simulink subsystem "rss_foc_controller_NewPlatform"  (R2023a)
settings: Solver=VariableStepAuto  StartTime=0.0  StopTime=10.0  RelTol=1e-3
undefined symbols (not defined in the file): Cdbl_tiFstTaskSmpTi, Cdbl_tiMedTaskSmpTi, Cdbl_tiSlwTaskSmpTi, ENM_AG_POS_EVAL_MODE, ENM_MOTO_STATUS, ENM_SYS_STATUS
(part 1 of 2)
settings Model: Creator=CAV2OFO  LastModifiedBy=xiaoqiang.yuan
settings SolverCC: AlgebraicLoopSolver=TrustRegion
settings OptimizationCC: ReuseModelBlockBuffer=off
settings DebuggingCC: UnconnectedInputMsg=warning  UnconnectedOutputMsg=warning  UnconnectedLineMsg=warning
settings ModelReferenceCC: EnableRefExpFcnMdlSchedulingChecks=on
settings RTWCC: DLArmComputeVersion=19.05

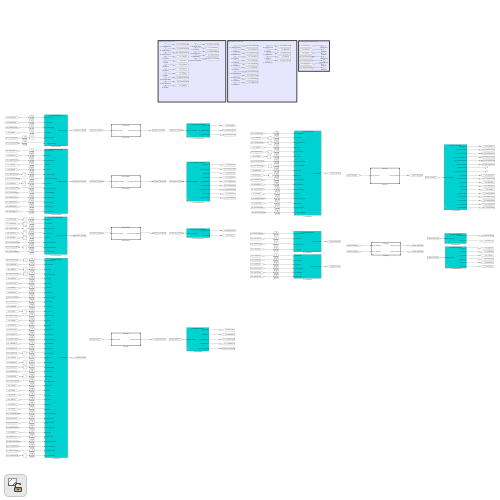
[thumbnail: Simulink's stored preview of the top-level diagram]
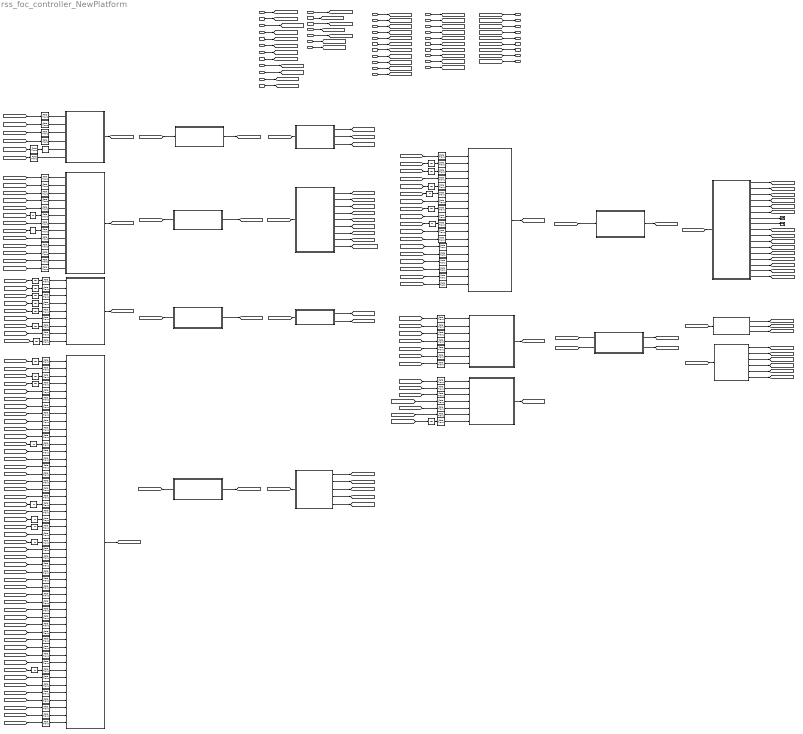
== system rss_foc_controller_NewPlatform ==
  note: Application software signals output
  note: Basic software signals input
  note: Communication signals input
  s16_nComRefMechSpd : Inport  OutDataTypeStr=dt_Standardize_s16p15b0
  u8_modeMCUOpMode : Inport  Port=2  OutDataTypeStr=uint8
  u16_ADSensActMechAg : Inport  Port=3  OutDataTypeStr=uint16
  u16_uADActPhCurr : Inport  Port=4  OutDataTypeStr=uint16
  u16_uADActPhCurrOfs : Inport  Port=5  OutDataTypeStr=uint16
  u8_numSectNum : Inport  Port=6  OutDataTypeStr=uint8
  u16_uADSplyVltg : Inport  Port=7  OutDataTypeStr=uint16
  u16_uADCtlBrdVltg : Inport  Port=8  OutDataTypeStr=uint16
  u16_uADGDVltg : Inport  Port=9  OutDataTypeStr=uint16
  bol_enPosSCDCalibEnFlg : Inport  Port=10  OutDataTypeStr=boolean
  u16_uADPwrTubTemp : Inport  Port=11  OutDataTypeStr=uint16
  u16_uADPCBTemp : Inport  Port=12  OutDataTypeStr=uint16
  u16_uADMotoTemp : Inport  Port=13  OutDataTypeStr=uint16
  u8_ctLossNoData : Inport  Port=14  OutDataTypeStr=uint8
  u8_ctComRolCnt : Inport  Port=15  OutDataTypeStr=uint8
  bol_flgHWOvrCurrFalt : Inport  Port=16  OutDataTypeStr=boolean
  bol_flgChipFalt : Inport  Port=17  OutDataTypeStr=boolean
  bol_flgPhiSensFalt : Inport  Port=18  OutDataTypeStr=boolean
  bol_enFaltInfoClrUDS14 : Inport  Port=19  OutDataTypeStr=boolean
  u16_vVehSpd : Inport  Port=20  OutDataTypeStr=fixdt(0,16,10^-2,0)
  u32_disOde : Inport  Port=21  OutDataTypeStr=fixdt(0,32,10^-1,0)
  u32_tiStamHi : Inport  Port=22  OutDataTypeStr=uint32
  u32_tiStamLo : Inport  Port=23  OutDataTypeStr=uint32
  u8_tOilTemp : Inport  Port=24  OutDataTypeStr=dt_Temp_u8p0bn40
  u8_psiOilFlow : Inport  Port=25  OutDataTypeStr=fixdt(0,8,5^-1,0)
  u8_psiUpLimOilFlow : Inport  Port=26  OutDataTypeStr=fixdt(0,8,5^-1,0)
  bol_flgBusOffFaltRaw : Inport  Port=27  OutDataTypeStr=boolean
  bol_flgFaltEnFlgUDS85 : Inport  Port=28  OutDataTypeStr=boolean
  bol_flgOvrTstCtlUDS2F : Inport  Port=29  OutDataTypeStr=boolean
  bol_flgWBSSt : Inport  Port=30  OutDataTypeStr=boolean
  bol_flgCRCFaltRaw : Inport  Port=31  OutDataTypeStr=boolean
  bol_flgMesgLngthFaltRaw : Inport  Port=32  OutDataTypeStr=boolean
  u8_FrzFrmSaveFlg : Inport  Port=33  OutDataTypeStr=uint8
  bol_flgSlepEn : Inport  Port=34  OutDataTypeStr=boolean
  bol_flgCrashFalt : Inport  Port=35  OutDataTypeStr=boolean
  bol_flgGDVltgHiLvl1 : Inport  Port=36  OutDataTypeStr=boolean
  bol_flgGDVltgLoLvl1 : Inport  Port=37  OutDataTypeStr=boolean
  u8_tMCUTemp : Inport  Port=38  OutDataTypeStr=dt_Temp_u8p0bn40
  u16_phiDvtSensElecAg : Inport  Port=39  OutDataTypeStr=dt_RadAng_u16r15b0
  bol_flgMosOpnCirFalt : Inport  Port=40  OutDataTypeStr=boolean
  ASW_AST : ModelReference  ModelNameDialog=ASW_AST.slx  SimulationMode=Normal  ModelReferenceVersion=6.236
  ASW_DcycGen : ModelReference  ModelNameDialog=ASW_DcycGen.slx  SimulationMode=Normal  ModelReferenceVersion=6.161
  ASW_OBD : ModelReference  ModelNameDialog=ASW_OBD.slx  SimulationMode=Normal  ModelReferenceVersion=6.308
  ASW_PhCurrGen : ModelReference  ModelNameDialog=ASW_PhCurrGen.slx  SimulationMode=Normal  ModelReferenceVersion=6.181
  ASW_PhVltgGen : ModelReference  ModelNameDialog=ASW_PhVltgGen.slx  SimulationMode=Normal  ModelReferenceVersion=6.211
  ASW_SigIn : ModelReference  ModelNameDialog=ASW_SigIn.slx  SimulationMode=Normal  ModelReferenceVersion=6.146
  Delay : Delay  DelayLength=1
  Delay1 : Delay  DelayLength=1
  Rate Transition{1,5..6,8,16,19,22,24..26,29..31,33,36,41,49,109} (18 alike) : RateTransition  Deterministic=off  OutPortSampleTime=round(double(Cdbl_tiMedTaskSmpTi),6)
  Rate Transition{2,9..10,14,48} (5 alike) : RateTransition  Deterministic=off  OutPortSampleTime=round(double(Cdbl_tiFstTaskSmpTi),8)
  Rate Transition100 : RateTransition  Deterministic=off  InitialCondition=ENM_AG_POS_EVAL_MODE.SENSORLESS  OutPortSampleTime=round(double(Cdbl_tiSlwTaskSmpTi),4)
  Rate Transition101 : RateTransition  Deterministic=off  InitialCondition=ENM_AG_POS_EVAL_MODE.SENSOR  OutPortSampleTime=round(double(Cdbl_tiSlwTaskSmpTi),4)
  Rate Transition{3..4,7,15,17..18,20..21,23,27..28,32,34..35,37..40,43..44,46..47,50..99,102..108} (79 alike) : RateTransition  Deterministic=off  OutPortSampleTime=round(double(Cdbl_tiSlwTaskSmpTi),4)
  Rate Transition11 : RateTransition  Deterministic=off  InitialCondition=ENM_MOTO_STATUS.OFF  OutPortSampleTime=round(double(Cdbl_tiFstTaskSmpTi),8)
  Rate Transition12 : RateTransition  Deterministic=off  InitialCondition=ENM_MOTO_STATUS.OFF  OutPortSampleTime=round(double(Cdbl_tiMedTaskSmpTi),6)
  Rate Transition13 : RateTransition  Deterministic=off  InitialCondition=ENM_AG_POS_EVAL_MODE.SENSORLESS  OutPortSampleTime=round(double(Cdbl_tiMedTaskSmpTi),6)
  Rate Transition42 : RateTransition  Deterministic=off  InitialCondition=ENM_MOTO_STATUS.OFF  OutPortSampleTime=round(double(Cdbl_tiSlwTaskSmpTi),4)
  Rate Transition45 : RateTransition  Deterministic=off  InitialCondition=ENM_MOTO_STATUS.OFF  OutPortSampleTime=round(double(Cdbl_tiSlwTaskSmpTi),4)
  Terminator11 : Terminator
  Terminator9 : Terminator
  Unit Delay : UnitDelay  InitialCondition=ENM_AG_POS_EVAL_MODE.SENSOR  SampleTime=-1  HasFrameUpgradeWarning=on
  Unit Delay{1..7,9..18,20..22} (20 alike) : UnitDelay  SampleTime=-1  HasFrameUpgradeWarning=on
  Unit Delay19 : UnitDelay  InitialCondition=ENM_MOTO_STATUS.OFF  SampleTime=-1  HasFrameUpgradeWarning=on
  Unit Delay32 : UnitDelay  InitialCondition=ENM_MOTO_STATUS.OFF  SampleTime=-1  HasFrameUpgradeWarning=on
  Unit Delay8 : UnitDelay  InitialCondition=ENM_SYS_STATUS.SYSINIT  SampleTime=-1  HasFrameUpgradeWarning=on
  sss_SigInSlwTaskIn : Subsystem  VariantControl=cstSenlCtrlLbl
  vrs_ASTSlwTaskIn : Subsystem  Variant=on  VariantControlMode=label  VariantControl=cstSenlCtrlLbl  LabelModeActiveChoice=cstHybrCtrlLbl
  vrs_ASTSlwTaskOut : Subsystem  Variant=on  VariantControlMode=label  VariantControl=Choice  LabelModeActiveChoice=cstHybrCtrlLbl
  vrs_DcycGenFstTaskIn : Subsystem  Variant=on  VariantControlMode=label  VariantControl=Choice  LabelModeActiveChoice=cstSensCtrlLbl
  vrs_DcycGenFstTaskOut : Subsystem  Variant=on  VariantControlMode=label  VariantControl=Choice  LabelModeActiveChoice=cstSensCtrlLbl
  vrs_OBDSlwTaskIn : Subsystem  Variant=on  VariantControlMode=label  VariantControl=cstSenlCtrlLbl  LabelModeActiveChoice=cstHybrCtrlLbl
  vrs_OBDSlwTaskOut : Subsystem  Variant=on  VariantControlMode=label  VariantControl=Choice  LabelModeActiveChoice=cstHybrCtrlLbl
  vrs_PhCurrGenSlwTaskIn : Subsystem  Variant=on  VariantControlMode=label  VariantControl=cstSenlCtrlLbl  LabelModeActiveChoice=cstHybrCtrlLbl
  vrs_PhCurrGenSlwTaskOut : Subsystem  Variant=on  VariantControlMode=label  VariantControl=Choice  LabelModeActiveChoice=cstSenlCtrlLbl
  vrs_PhVltgGenMedTaskIn : Subsystem  Variant=on  VariantControlMode=label  VariantControl=Choice  LabelModeActiveChoice=cstHybrCtrlLbl
  vrs_PhVltgGenMedTaskOut : Subsystem  Variant=on  VariantControlMode=label  VariantControl=Choice  LabelModeActiveChoice=cstHybrCtrlLbl
  vrs_SigInMedTaskIn : Subsystem  Variant=on  VariantControlMode=label  VariantControl=cstSenlCtrlLbl  LabelModeActiveChoice=cstSensCtrlLbl
  vrs_SigInMedTaskOut : Subsystem  Variant=on  VariantControlMode=label  VariantControl=Choice  LabelModeActiveChoice=cstSensCtrlLbl
  vrs_SigInSlwTaskOut : Subsystem  Variant=on  VariantControlMode=label  VariantControl=Choice  LabelModeActiveChoice=cstSenlCtrlLbl
  genXYZDutyCycl : Outport
  enmMotStas : Outport  Port=2
  enmSysStas : Outport  Port=3
  bolCalibSuccFlag : Outport  Port=4
  arSensErrMechAng : Outport  Port=5
  iEstSplyCurr : Outport  Port=6
  iActLineCurr : Outport  Port=7
  u16_phiSensElecAgDvt : Outport  Port=8
  s16_nActElecSpdComFlt : Outport  Port=9
  wires:
  u16_ADSensActMechAg/1 -> [u16_ADSensActMechAg]
  u16_uADActPhCurr/1 -> [u16_uADActPhCurr]
  u16_uADSplyVltg/1 -> [u16_uADSplyVltg]
  [u16_dcycPhDyc] -> genXYZDutyCycl/1
  s16_nComRefMechSpd/1 -> [s16_nComRefMechSpd]
  [s16_iEstSplyCurr] -> iEstSplyCurr/1
  [s16_ampActPhCurrAmp] -> iActLineCurr/1
  [u16_phiModulActElecAg] -> Unit Delay4/1
  [s16_nPredActElecSpd] -> Rate Transition14/1
  [u16_ampDycAmp] -> Rate Transition2/1
  [enm_stMotoSt] -> Rate Transition11/1
  [u16_phiDaxQaxVltgAg] -> Rate Transition10/1
  Rate Transition14/1 -> Delay1/1
  [s16_nActElecSpd] -> Unit Delay5/1
  [s16_nRefElecSpd] -> Unit Delay7/1
  [s16_trqRefTqLim] -> Unit Delay12/1
  [u16_dcycPhDyc] -> Delay/1
  Delay/1 -> Rate Transition31/1
  vrs_PhVltgGenMedTaskIn/1(busPhVltgGen_MedTaskIn) -> [busPhVltgGen_MedTaskIn]
  Rate Transition25/1 -> vrs_PhVltgGenMedTaskIn/1(s16_iRefDaxQaxCurr)
  Rate Transition26/1 -> vrs_PhVltgGenMedTaskIn/2(s16_iActPhCurr)
  Rate Transition1/1 -> vrs_PhVltgGenMedTaskIn/3(u16_phiSensActElecAg)
  Rate Transition6/1 -> vrs_PhVltgGenMedTaskIn/4(u16_uSplyVltg)
  Rate Transition12/1 -> vrs_PhVltgGenMedTaskIn/5(enm_stMotoSt)
  Rate Transition29/1 -> vrs_PhVltgGenMedTaskIn/6(u16_phiModulActElecAg)
  [busPhVltgGen_MedTaskOut] -> vrs_PhVltgGenMedTaskOut/1(busPhVltgGen_MedTaskOut)
  vrs_PhVltgGenMedTaskOut/2(u16_phiDaxQaxVltgAg) -> [u16_phiDaxQaxVltgAg]
  vrs_PhVltgGenMedTaskOut/3(u16_phiActElecAg) -> [u16_phiActElecAg]
  vrs_PhVltgGenMedTaskOut/1(u16_ampDycAmp) -> [u16_ampDycAmp]
  vrs_PhVltgGenMedTaskOut/4(s16_nActElecSpd) -> [s16_nActElecSpd]
  vrs_PhVltgGenMedTaskOut/7(s16_uModulDaxQaxVltg) -> [s16_uModulDaxQaxVltg]
  vrs_PhVltgGenMedTaskOut/5(s16_iActDaxQaxCurr) -> [s16_iActDaxQaxCurr]
  vrs_PhVltgGenMedTaskOut/6(s16_nPredActElecSpd) -> [s16_nPredActElecSpd]
  Rate Transition2/1 -> vrs_DcycGenFstTaskIn/1(u16_ampDycAmp)
  Rate Transition9/1 -> vrs_DcycGenFstTaskIn/2(u16_phiActElecAg)
  Rate Transition10/1 -> vrs_DcycGenFstTaskIn/3(u16_phiDaxQaxVltgAg)
  Rate Transition11/1 -> vrs_DcycGenFstTaskIn/4(enm_stMotoSt)
  Delay1/1 -> vrs_DcycGenFstTaskIn/5(s16_nPredActElecSpd)
  vrs_DcycGenFstTaskIn/1(busDcycGen_FstTaskIn) -> [busDcycGen_FstTaskIn]
  [busDcycGen_FstTaskOut] -> vrs_DcycGenFstTaskOut/1(busDcycGen_FstTaskOut)
  vrs_DcycGenFstTaskOut/1(u16_dcycPhDyc) -> [u16_dcycPhDyc]
  vrs_DcycGenFstTaskOut/2(u16_ampMaxNrmVltgAmp) -> [u16_ampMaxNrmVltgAmp]
  vrs_DcycGenFstTaskOut/3(u16_phiModulActElecAg) -> [u16_phiModulActElecAg]
  vrs_PhCurrGenSlwTaskOut/1(s16_iRefDaxQaxCurr) -> [s16_iRefDaxQaxCurr]
  bol_enPosSCDCalibEnFlg/1 -> [bol_enPosSCDCalibEnFlg]
  Unit Delay4/1 -> Rate Transition29/1
  Unit Delay5/1 -> Rate Transition18/1
  [s16_nRmpRefElecSpd] -> Unit Delay11/1
  [bol_enPosSCDCalibEnFlg] -> Rate Transition39/1
  [bol_flgShOffFlg] -> Unit Delay13/1
  vrs_PhCurrGenSlwTaskOut/2(enm_stMotoSt) -> [enm_stMotoSt]
  vrs_ASTSlwTaskOut/10(s16_nRmpRefElecSpd) -> [s16_nRmpRefElecSpd]
  vrs_ASTSlwTaskOut/3(s16_trqPosSCDCalibRefTq) -> [s16_trqPosSCDCalibRefTq]
  vrs_ASTSlwTaskOut/2(s16_ampActPhCurrAmp) -> [s16_ampActPhCurrAmp]
  vrs_ASTSlwTaskOut/6(u16_ADSensMechAgDvt) -> [u16_ADSensMechAgDvt]
  vrs_ASTSlwTaskOut/8(bol_flgPosSCDCalibPermFail) -> Terminator11/1
  vrs_ASTSlwTaskOut/9(s16_trqRefTqLim) -> [s16_trqRefTqLim]
  vrs_ASTSlwTaskOut/4(u16_phiPosSCDCalibElecAg) -> [u16_phiPosSCDCalibElecAg]
  vrs_ASTSlwTaskOut/5(bol_flgPosSCDCalibSucFlg) -> [bol_flgPosSCDCalibSucFlg]
  vrs_ASTSlwTaskOut/7(enm_stPosSCDCalibSt) -> Terminator9/1
  vrs_ASTSlwTaskOut/1(s16_iEstSplyCurr) -> [s16_iEstSplyCurr]
  [busPhCurrGen_SlwTaskOut] -> vrs_PhCurrGenSlwTaskOut/1(busMotoCtl_SlwTaskOut)
  ASW_AST/1 -> [busAST_SlwTaskOut]
  [busAST_SlwTaskIn] -> ASW_AST/1
  [busAST_SlwTaskOut] -> vrs_ASTSlwTaskOut/1(busAST_SlwTaskOut)
  [s16_iActDaxQaxCurr] -> Unit Delay9/1
  [s16_uModulDaxQaxVltg] -> Unit Delay10/1
  [s16_nComRefMechSpd] -> Rate Transition4/1
  [s16_nActElecSpd] -> Unit Delay6/1
  Unit Delay6/1 -> Rate Transition15/1
  Unit Delay9/1 -> Rate Transition40/1
  Unit Delay10/1 -> Rate Transition23/1
  Unit Delay11/1 -> Rate Transition20/1
  Unit Delay12/1 -> Rate Transition21/1
  [s16_nRmpRefElecSpd] -> Unit Delay3/1
  [busOBD_SlwTaskIn] -> ASW_OBD/1
  [enm_stMotoSt] -> Unit Delay19/1
  [s16_nActElecSpd] -> Rate Transition44/1
  [busOBD_SlwTaskOut] -> vrs_OBDSlwTaskOut/1(busOBD_SlwTaskOut)
  ASW_OBD/1 -> [busOBD_SlwTaskOut]
  vrs_SigInMedTaskOut/1(u16_phiSensActElecAg) -> [u16_phiSensActElecAg]
  ASW_SigIn/1 -> [busSigIn_MedTaskOut]
  [busSigIn_MedTaskOut] -> vrs_SigInMedTaskOut/1(busSigIn_MedTaskOut)
  [busSigIn_MedTaskIn] -> ASW_SigIn/1
  [u16_ADSensActMechAg] -> Rate Transition49/1
  vrs_ASTSlwTaskOut/11(bol_flgShOffFlg) -> [bol_flgShOffFlg]
  Unit Delay13/1 -> Rate Transition38/1
  [bol_enPosSCDCalibEnFlg] -> Rate Transition48/1
  [u16_phiSensActElecAg] -> Unit Delay15/1
  Unit Delay15/1 -> Rate Transition51/1
  Rate Transition36/1 -> vrs_PhVltgGenMedTaskIn/7(u16_phiPosSCDCalibElecAg)
  Rate Transition31/1 -> vrs_PhVltgGenMedTaskIn/8(u16_dcycPhDyc)
  Rate Transition41/1 -> vrs_PhVltgGenMedTaskIn/9(bol_enPosSCDCalibEnFlg)
  Rate Transition13/1 -> vrs_PhVltgGenMedTaskIn/10(enm_modeAgEvalMode)
  Rate Transition33/1 -> vrs_PhVltgGenMedTaskIn/11(s16_nRmpRefElecSpd)
  [s16_trqPosSCDCalibRefTq] -> Unit Delay16/1
  Unit Delay16/1 -> Rate Transition53/1
  vrs_ASTSlwTaskOut/12(s16_nRefElecSpd) -> [s16_nRefElecSpd]
  [enm_stMotoSt] -> Unit Delay32/1
  Unit Delay7/1 -> Rate Transition17/1
  u16_uADPwrTubTemp/1 -> [u16_uADPwrTubTemp]
  u16_uADPCBTemp/1 -> [u16_uADPCBTemp]
  u16_uADMotoTemp/1 -> [u16_uADMotoTemp]
  u8_ctLossNoData/1 -> [u8_ctLossNoData]
  u8_ctComRolCnt/1 -> [u8_ctComRolCnt]
  u8_modeMCUOpMode/1 -> [u8_modeMCUOpMode]
  [u16_uADActPhCurr] -> Rate Transition22/1
  [u16_uADPwrTubTemp] -> Rate Transition61/1
  [u16_uADPCBTemp] -> Rate Transition62/1
  [u16_uADMotoTemp] -> Rate Transition63/1
  Rate Transition61/1 -> sss_SigInSlwTaskIn/3(u16_uADPwrTubTemp)
  Rate Transition62/1 -> sss_SigInSlwTaskIn/4(u16_uADPCBTemp)
  Rate Transition63/1 -> sss_SigInSlwTaskIn/5(u16_uADMotoTemp)
  sss_SigInSlwTaskIn/1(busSigIn_SlowTaskInp) -> [busSigIn_SlwTaskIn]
  [busSigIn_SlwTaskIn] -> ASW_SigIn/2
  ASW_SigIn/2 -> [busSigIn_SlwTaskOut]
  vrs_SigInMedTaskOut/2(s16_iActPhCurr) -> [s16_iActPhCurr]
  [busSigIn_SlwTaskOut] -> vrs_SigInSlwTaskOut/1(busSigIn_SlwTaskOut)
  vrs_SigInSlwTaskOut/4(u8_tPCBTemp) -> [u8_tPCBTemp]
  vrs_SigInSlwTaskOut/5(u8_tMotoTemp) -> [u8_tMotoTemp]
  vrs_OBDSlwTaskOut/1(busOBD_FaltSt) -> [busOBD_FaltSt]
  vrs_OBDSlwTaskOut/2(u8_stMaxFaltLvl) -> [u8_stMaxFaltLvl]
  vrs_OBDSlwTaskOut/3(s16_nFaltRefMechSpd) -> [s16_nFaltRefMechSpd]
  vrs_OBDSlwTaskOut/4(s16_trqFaltRefTqLim) -> [s16_trqFaltRefTqLim]
  [s16_ampActPhCurrAmp] -> Unit Delay17/1
  [u16_uSplyVltg] -> Rate Transition65/1
  [u8_tPwrTubTemp] -> Rate Transition66/1
  [u8_tPCBTemp] -> Rate Transition67/1
  [u8_tMotoTemp] -> Rate Transition68/1
  [u8_ctLossNoData] -> Rate Transition69/1
  [u8_ctComRolCnt] -> Rate Transition70/1
  vrs_ASTSlwTaskOut/13(enm_stSysSt) -> [enm_stSysSt]
  [busOBD_FaltSt] -> Unit Delay1/1
  Unit Delay1/1 -> Rate Transition73/1
  Unit Delay3/1 -> Rate Transition43/1
  Unit Delay17/1 -> Rate Transition64/1
  [enm_stMotoSt] -> enmMotStas/1
  [enm_stSysSt] -> enmSysStas/1
  [bol_flgPosSCDCalibSucFlg] -> bolCalibSuccFlag/1
  [u16_ADSensMechAgDvt] -> arSensErrMechAng/1
  [s16_nRmpRefElecSpd] -> Rate Transition33/1
  Rate Transition19/1 -> vrs_PhVltgGenMedTaskIn/13(u16_ampMaxNrmVltgAmp)
  [u16_uADActPhCurrOfs] -> Rate Transition24/1
  [u8_numSectNum] -> Rate Transition30/1
  u16_uADActPhCurrOfs/1 -> [u16_uADActPhCurrOfs]
  u8_numSectNum/1 -> [u8_numSectNum]
  vrs_SigInSlwTaskOut/3(u8_tPwrTubTemp) -> [u8_tPwrTubTemp]
  [u16_phiActElecAg] -> Rate Transition9/1
  [u16_uCtlBrdVltg] -> Rate Transition27/1
  vrs_SigInSlwTaskOut/1(u16_uCtlBrdVltg) -> [u16_uCtlBrdVltg]
  Rate Transition28/1 -> sss_SigInSlwTaskIn/1(u16_uADCtlBrdVltg)
  [u16_uADCtlBrdVltg] -> Rate Transition28/1
  u16_uADCtlBrdVltg/1 -> [u16_uADCtlBrdVltg]
  [busDcycGen_FstTaskIn] -> ASW_DcycGen/1
  [busPhVltgGen_MedTaskIn] -> ASW_PhVltgGen/1
  [busPhCurrGen_SlwTaskIn] -> ASW_PhCurrGen/1
  ASW_DcycGen/1 -> [busDcycGen_FstTaskOut]
  ASW_PhVltgGen/1 -> [busPhVltgGen_MedTaskOut]
  ASW_PhCurrGen/1 -> [busPhCurrGen_SlwTaskOut]
  u16_uADGDVltg/1 -> [u16_uADGDVltg]
  Rate Transition32/1 -> sss_SigInSlwTaskIn/2(u16_uADGDVltg)
  [u16_uADGDVltg] -> Rate Transition32/1
  vrs_SigInSlwTaskOut/2(u16_uGDVltg) -> [u16_uGDVltg]
  [enm_stSysSt] -> Unit Delay8/1
  [bol_flgHWOvrCurrFalt] -> Rate Transition46/1
  [bol_flgChipFalt] -> Rate Transition52/1
  [bol_flgPhiSensFalt] -> Rate Transition54/1
  [u16_uADActPhCurr] -> Rate Transition55/1
  [u16_uADPwrTubTemp] -> Rate Transition56/1
  [u16_uADPCBTemp] -> Rate Transition57/1
  [u16_uADMotoTemp] -> Rate Transition58/1
  [s16_pwrSplyElecPwr] -> Unit Delay2/1
  bol_flgHWOvrCurrFalt/1 -> [bol_flgHWOvrCurrFalt]
  bol_flgChipFalt/1 -> [bol_flgChipFalt]
  bol_flgPhiSensFalt/1 -> [bol_flgPhiSensFalt]
  vrs_ASTSlwTaskOut/14(s16_pwrSplyElecPwr) -> [s16_pwrSplyElecPwr]
  Unit Delay2/1 -> Rate Transition59/1
  Unit Delay8/1 -> Rate Transition34/1
  [s16_iActPhCurr] -> Rate Transition60/1
  [s16_iEstSplyCurr] -> Unit Delay14/1
  [s16_iRefDaxQaxCurr] -> Unit Delay20/1
  [s16_iActDaxQaxCurr] -> Rate Transition81/1
  [bol_flgShOffFlg] -> Unit Delay18/1
  Unit Delay14/1 -> Rate Transition71/1
  Unit Delay18/1 -> Rate Transition82/1
  [bol_enFaltInfoClrUDS14] -> Rate Transition83/1
  [u16_vVehSpd] -> Rate Transition84/1
  [u32_disOde] -> Rate Transition85/1
  [u32_tiStamHi] -> Rate Transition86/1
  [u32_tiStamLo] -> Rate Transition87/1
  [u8_psiOilFlow] -> Rate Transition88/1
  [u8_tOilTemp] -> Rate Transition89/1
  [bol_enPosSCDCalibEnFlg] -> Rate Transition90/1
  [u8_psiUpLimOilFlow] -> Rate Transition91/1
  bol_enFaltInfoClrUDS14/1 -> [bol_enFaltInfoClrUDS14]
  u16_vVehSpd/1 -> [u16_vVehSpd]
  u32_disOde/1 -> [u32_disOde]
  u32_tiStamHi/1 -> [u32_tiStamHi]
  u32_tiStamLo/1 -> [u32_tiStamLo]
  u8_tOilTemp/1 -> [u8_tOilTemp]
  u8_psiOilFlow/1 -> [u8_psiOilFlow]
  u8_psiUpLimOilFlow/1 -> [u8_psiUpLimOilFlow]
  bol_flgBusOffFaltRaw/1 -> [bol_flgBusOffFaltRaw]
  bol_flgFaltEnFlgUDS85/1 -> [bol_flgFaltEnFlgUDS85]
  bol_flgOvrTstCtlUDS2F/1 -> [bol_flgOvrTstCtlUDS2F]
  bol_flgWBSSt/1 -> [bol_flgWBSSt]
  [bol_flgBusOffFaltRaw] -> Rate Transition93/1
  [bol_flgFaltEnFlgUDS85] -> Rate Transition94/1
  [bol_flgWBSSt] -> Rate Transition95/1
  bol_flgCRCFaltRaw/1 -> [bol_flgCRCFaltRaw]
  bol_flgMesgLngthFaltRaw/1 -> [bol_flgMesgLngthFaltRaw]
  [bol_flgCRCFaltRaw] -> Rate Transition96/1
  [bol_flgMesgLngthFaltRaw] -> Rate Transition97/1
  [s16_nComRefMechSpd] -> Rate Transition98/1
  vrs_PhVltgGenMedTaskOut/8(u16_psiEstPermMagFlx) -> [u16_psiEstPermMagFlx]
  [u16_psiEstPermMagFlx] -> Rate Transition99/1
  Rate Transition43/1 -> vrs_OBDSlwTaskIn/1(s16_nRmpRefElecSpd)
  Rate Transition44/1 -> vrs_OBDSlwTaskIn/2(s16_nActElecSpd)
  Rate Transition45/1 -> vrs_OBDSlwTaskIn/3(enm_stMotoSt)
  Rate Transition64/1 -> vrs_OBDSlwTaskIn/4(s16_ampActPhCurrAmp)
  Rate Transition65/1 -> vrs_OBDSlwTaskIn/5(u16_uSplyVltg)
  Rate Transition66/1 -> vrs_OBDSlwTaskIn/6(u8_tPwrTubTemp)
  Rate Transition67/1 -> vrs_OBDSlwTaskIn/7(u8_tPCBTemp)
  Rate Transition68/1 -> vrs_OBDSlwTaskIn/8(u8_tMotoTemp)
  Rate Transition69/1 -> vrs_OBDSlwTaskIn/9(u8_ctLossNoData)
  Rate Transition70/1 -> vrs_OBDSlwTaskIn/10(u8_ctComRolCnt)
  Rate Transition27/1 -> vrs_OBDSlwTaskIn/11(u16_uCtlBrdVltg)
  Rate Transition34/1 -> vrs_OBDSlwTaskIn/12(enm_stSysSt)
  Rate Transition46/1 -> vrs_OBDSlwTaskIn/13(bol_flgHWOvrCurrFalt)
  Rate Transition52/1 -> vrs_OBDSlwTaskIn/14(bol_flgChipFalt)
  Rate Transition54/1 -> vrs_OBDSlwTaskIn/15(bol_flgPhiSensFalt)
  Rate Transition55/1 -> vrs_OBDSlwTaskIn/16(u16_uADActPhCurr)
  Rate Transition56/1 -> vrs_OBDSlwTaskIn/17(u16_uADPwrTubTemp)
  Rate Transition57/1 -> vrs_OBDSlwTaskIn/18(u16_uADPCBTemp)
  Rate Transition58/1 -> vrs_OBDSlwTaskIn/19(u16_uADMotoTemp)
  Rate Transition59/1 -> vrs_OBDSlwTaskIn/20(s16_pwrSplyElecPwr)
  Rate Transition60/1 -> vrs_OBDSlwTaskIn/21(s16_iActPhCurr)
  Rate Transition71/1 -> vrs_OBDSlwTaskIn/22(s16_iEstSplyCurr)
  Rate Transition80/1 -> vrs_OBDSlwTaskIn/23(s16_iRefDaxQaxCurr)
  Rate Transition81/1 -> vrs_OBDSlwTaskIn/24(s16_iActDaxQaxCurr)
  Rate Transition82/1 -> vrs_OBDSlwTaskIn/25(bol_flgShOffFlg)
  Rate Transition83/1 -> vrs_OBDSlwTaskIn/26(bol_enFaltInfoClrUDS14)
  Rate Transition84/1 -> vrs_OBDSlwTaskIn/27(u16_vVehSpd)
  Rate Transition85/1 -> vrs_OBDSlwTaskIn/28(u32_disOde)
  Rate Transition86/1 -> vrs_OBDSlwTaskIn/29(u32_tiStamHi)
  Rate Transition87/1 -> vrs_OBDSlwTaskIn/30(u32_tiStamLo)
  Rate Transition88/1 -> vrs_OBDSlwTaskIn/31(u8_psiOilFlow)
  Rate Transition89/1 -> vrs_OBDSlwTaskIn/32(u8_tOilTemp)
  Rate Transition90/1 -> vrs_OBDSlwTaskIn/33(bol_enPosSCDCalibEnFlg)
  Rate Transition91/1 -> vrs_OBDSlwTaskIn/34(u8_psiUpLimOilFlow)
  Rate Transition93/1 -> vrs_OBDSlwTaskIn/35(bol_flgBusOffFaltRaw)
  Rate Transition94/1 -> vrs_OBDSlwTaskIn/36(bol_flgFaltEnFlgUDS85)
  Rate Transition95/1 -> vrs_OBDSlwTaskIn/37(bol_flgWBSSt)
  Rate Transition96/1 -> vrs_OBDSlwTaskIn/38(bol_flgCRCFaltRaw)
  Rate Transition97/1 -> vrs_OBDSlwTaskIn/39(bol_flgMesgLngthFaltRaw)
  Rate Transition98/1 -> vrs_OBDSlwTaskIn/40(s16_nComRefMechSpd)
  Rate Transition99/1 -> vrs_OBDSlwTaskIn/41(u16_psiEstPermMagFlx)
  vrs_OBDSlwTaskIn/1(busSlowTaskInp) -> [busOBD_SlwTaskIn]
  Rate Transition49/1 -> vrs_SigInMedTaskIn/1(u16_ADSensActMechAg)
  Rate Transition22/1 -> vrs_SigInMedTaskIn/2(u16_uADActPhCurr)
  Rate Transition24/1 -> vrs_SigInMedTaskIn/3(u16_uADActPhCurrOfs)
  Rate Transition30/1 -> vrs_SigInMedTaskIn/4(u8_numSectNum)
  vrs_SigInMedTaskIn/1(busSigIn_MedTaskIn) -> [busSigIn_MedTaskIn]
  vrs_ASTSlwTaskOut/15(enm_modeAgEvalMode) -> [enm_modeAgEvalMode]
  Rate Transition17/1 -> vrs_PhCurrGenSlwTaskIn/1(s16_nRefElecSpd)
  Rate Transition18/1 -> vrs_PhCurrGenSlwTaskIn/2(s16_nActElecSpd)
  Rate Transition20/1 -> vrs_PhCurrGenSlwTaskIn/3(s16_nRmpRefElecSpd)
  Rate Transition21/1 -> vrs_PhCurrGenSlwTaskIn/4(s16_trqRefTqLim)
  Rate Transition38/1 -> vrs_PhCurrGenSlwTaskIn/5(bol_flgShOffFlg)
  Rate Transition39/1 -> vrs_PhCurrGenSlwTaskIn/6(bol_enPosSCDCalibEnFlg)
  Rate Transition53/1 -> vrs_PhCurrGenSlwTaskIn/7(s16_trqPosSCDCalibRefTq)
  vrs_PhCurrGenSlwTaskIn/1(busPhCurrGen_SlwTaskIn) -> [busPhCurrGen_SlwTaskIn]
  Rate Transition4/1 -> vrs_ASTSlwTaskIn/1(s16_nComRefMechSpd)
  Rate Transition15/1 -> vrs_ASTSlwTaskIn/2(s16_nActElecSpd)
  Rate Transition23/1 -> vrs_ASTSlwTaskIn/3(s16_uModulDaxQaxVltg)
  Rate Transition37/1 -> vrs_ASTSlwTaskIn/4(u16_uSplyVltg)
  Rate Transition40/1 -> vrs_ASTSlwTaskIn/5(s16_iActDaxQaxCurr)
  Rate Transition42/1 -> vrs_ASTSlwTaskIn/6(enm_stMotoSt)
  Rate Transition47/1 -> vrs_ASTSlwTaskIn/7(bol_enPosSCDCalibEnFlg)
  Rate Transition51/1 -> vrs_ASTSlwTaskIn/8(u16_phiSensActElecAg)
  Rate Transition72/1 -> vrs_ASTSlwTaskIn/9(u8_stMaxFaltLvl)
  Rate Transition73/1 -> vrs_ASTSlwTaskIn/10(busOBD_FaltSt)
  Rate Transition74/1 -> vrs_ASTSlwTaskIn/11(s16_nFaltRefMechSpd)
  Rate Transition75/1 -> vrs_ASTSlwTaskIn/12(s16_trqFaltRefTqLim)
  Rate Transition79/1 -> vrs_ASTSlwTaskIn/13(u8_modeMCUOpMode)
  Rate Transition3/1 -> vrs_ASTSlwTaskIn/14(u8_tPCBTempSubs)
  Rate Transition92/1 -> vrs_ASTSlwTaskIn/15(bol_flgOvrTstCtlUDS2F)
  vrs_ASTSlwTaskIn/1(busAST_SlwTaskIn) -> [busAST_SlwTaskIn]
  Rate Transition100/1 -> vrs_PhCurrGenSlwTaskIn/8(enm_modeAgEvalMode)
  [enm_modeAgEvalMode] -> Rate Transition100/1
  Rate Transition101/1 -> vrs_OBDSlwTaskIn/42(enm_modeAgEvalMode)
  [enm_modeAgEvalMode] -> Unit Delay/1
  vrs_OBDSlwTaskOut/5(bol_flgPhiSensFaltRawFlg) -> [bol_flgPhiSensFaltRawFlg]
  Rate Transition102/1 -> vrs_ASTSlwTaskIn/16(bol_flgPhiSensFaltRawFlg)
  Unit Delay/1 -> Rate Transition101/1
  Rate Transition48/1 -> vrs_DcycGenFstTaskIn/6(bol_enPosSCDCalibEnFlg)
  [bol_enPosSCDCalibEnFlg] -> Rate Transition41/1
  [u16_phiPosSCDCalibElecAg] -> Rate Transition36/1
  [enm_stMotoSt] -> Rate Transition12/1
  [u16_uSplyVltg] -> Rate Transition6/1
  [u16_phiSensActElecAg] -> Rate Transition1/1
  [s16_iActPhCurr] -> Rate Transition26/1
  [s16_iRefDaxQaxCurr] -> Rate Transition25/1
  [enm_modeAgEvalMode] -> Rate Transition13/1
  [u16_uSplyVltg] -> Rate Transition37/1
  Unit Delay32/1 -> Rate Transition42/1
  [bol_enPosSCDCalibEnFlg] -> Rate Transition47/1
  [u8_stMaxFaltLvl] -> Rate Transition72/1
  [s16_nFaltRefMechSpd] -> Rate Transition74/1
  [s16_trqFaltRefTqLim] -> Rate Transition75/1
  [u8_modeMCUOpMode] -> Rate Transition79/1
  [u8_tPCBTempSubs] -> Rate Transition3/1
  [bol_flgOvrTstCtlUDS2F] -> Rate Transition92/1
  [bol_flgPhiSensFaltRawFlg] -> Rate Transition102/1
  Unit Delay19/1 -> Rate Transition45/1
  Unit Delay20/1 -> Rate Transition80/1
  [u8_FrzFrmSaveFlg] -> Rate Transition76/1
  Rate Transition76/1 -> vrs_ASTSlwTaskIn/17(u8_FrzFrmSaveFlg)
  u8_FrzFrmSaveFlg/1 -> [u8_FrzFrmSaveFlg]
  [bol_flgSlepEn] -> Rate Transition77/1
  Rate Transition77/1 -> vrs_ASTSlwTaskIn/18(bol_flgSlepEn)
  bol_flgSlepEn/1 -> [bol_flgSlepEn]
  [bol_flgCrashFalt] -> Rate Transition78/1
  Rate Transition78/1 -> vrs_OBDSlwTaskIn/43(bol_flgCrashFalt)
  [bol_flgGDVltgHiLvl1] -> Rate Transition103/1
  Rate Transition103/1 -> vrs_OBDSlwTaskIn/44(bol_flgGDVltgHiLvl1)
  Rate Transition104/1 -> vrs_OBDSlwTaskIn/45(bol_flgGDVltgLoLvl1)
  [bol_flgGDVltgLoLvl1] -> Rate Transition104/1
  bol_flgCrashFalt/1 -> [bol_flgCrashFalt]
  bol_flgGDVltgHiLvl1/1 -> [bol_flgGDVltgHiLvl1]
  bol_flgGDVltgLoLvl1/1 -> [bol_flgGDVltgLoLvl1]
  [u8_tMCUTemp] -> Rate Transition50/1
  Rate Transition50/1 -> vrs_OBDSlwTaskIn/46(u8_tMCUTemp)
  u8_tMCUTemp/1 -> [u8_tMCUTemp]
  [u8_tMCUTemp] -> Rate Transition105/1
  Unit Delay21/1 -> Rate Transition106/1
  [busOBD_FaltSt] -> Unit Delay21/1
  Rate Transition105/1 -> sss_SigInSlwTaskIn/6(u8_tMCUTemp)
  Rate Transition106/1 -> sss_SigInSlwTaskIn/7(busOBD_FaltSt)
  vrs_SigInSlwTaskOut/6(u8_tPCBTempSubs) -> [u8_tPCBTempSubs]
  [u8_tPCBTempSubs] -> Rate Transition107/1
  Rate Transition107/1 -> vrs_OBDSlwTaskIn/47(u8_tPCBTempSubs)
  [u16_uGDVltg] -> Rate Transition108/1
  Rate Transition108/1 -> vrs_OBDSlwTaskIn/48(u16_uGDVltg)
  [u8_tPCBTempSubs] -> Rate Transition109/1
  Rate Transition109/1 -> vrs_PhVltgGenMedTaskIn/12(u8_tPCBTempSubs)
  [u16_ampMaxNrmVltgAmp] -> Rate Transition19/1
  vrs_SigInMedTaskOut/3(u16_uSplyVltg) -> [u16_uSplyVltg]
  Rate Transition5/1 -> vrs_SigInMedTaskIn/5(u16_uADSplyVltg)
  [u16_uADSplyVltg] -> Rate Transition5/1
  vrs_PhVltgGenMedTaskOut/9(s16_phiOpnLpAgClsLpAgDvt) -> [s16_phiOpnLpAgClsLpAgDvt]
  Rate Transition7/1 -> vrs_PhCurrGenSlwTaskIn/9(s16_phiOpnLpAgClsLpAgDvt)
  [s16_phiOpnLpAgClsLpAgDvt] -> Unit Delay22/1
  Unit Delay22/1 -> Rate Transition7/1
  vrs_ASTSlwTaskOut/16(u16_phiSensElecAgDvt) -> [u16_phiSensElecAgDvt]
  [u16_phiSensElecAgDvt] -> u16_phiSensElecAgDvt/1
  vrs_ASTSlwTaskOut/17(s16_nActElecSpdComFlt) -> [s16_nActElecSpdComFlt]
  [s16_nActElecSpdComFlt] -> s16_nActElecSpdComFlt/1
  Rate Transition8/1 -> vrs_SigInMedTaskIn/6(u16_phiDvtSensElecAg)
  [u16_phiDvtSensElecAg] -> Rate Transition8/1
  Rate Transition16/1 -> vrs_SigInMedTaskIn/7(bol_enPosSCDCalibEnFlg)
  [bol_enPosSCDCalibEnFlg] -> Rate Transition16/1
  u16_phiDvtSensElecAg/1 -> [u16_phiDvtSensElecAg]
  [bol_flgMosOpnCirFalt] -> Rate Transition35/1
  Rate Transition35/1 -> vrs_OBDSlwTaskIn/49(bol_flgMosOpnCirFalt)
  bol_flgMosOpnCirFalt/1 -> [bol_flgMosOpnCirFalt]

== system rss_foc_controller_NewPlatform/sss_SigInSlwTaskIn ==
  u16_uADCtlBrdVltg : Inport
  u16_uADGDVltg : Inport  Port=2
  u16_uADPwrTubTemp : Inport  Port=3
  u16_uADPCBTemp : Inport  Port=4
  u16_uADMotoTemp : Inport  Port=5
  u8_tMCUTemp : Inport  Port=6
  busOBD_FaltSt : Inport  Port=7
  Bus Creator : BusCreator  Inputs=7  OutDataTypeStr=Bus: BUS_SIGIN_SLW_TASK_IN
      settings: InheritFromInputs=off
  busSigIn_SlowTaskInp : Outport  OutDataTypeStr=Bus: BUS_SIGIN_SLW_TASK_IN
  wires:
  busOBD_FaltSt/1 -> Bus Creator/7
  u8_tMCUTemp/1 -> Bus Creator/6
  u16_uADMotoTemp/1 -> Bus Creator/5
  u16_uADPCBTemp/1 -> Bus Creator/4
  u16_uADPwrTubTemp/1 -> Bus Creator/3
  u16_uADGDVltg/1 -> Bus Creator/2
  u16_uADCtlBrdVltg/1 -> Bus Creator/1
  Bus Creator/1 -> busSigIn_SlowTaskInp/1

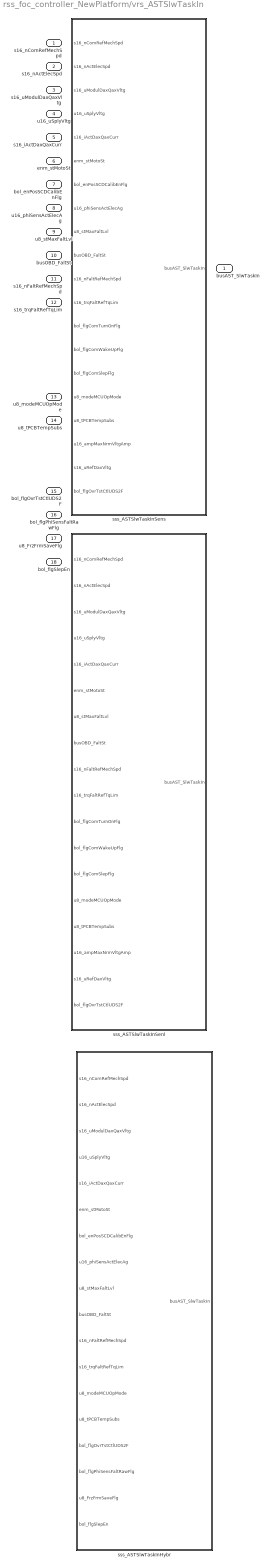
== system rss_foc_controller_NewPlatform/vrs_ASTSlwTaskIn ==
  s16_nComRefMechSpd : Inport
  s16_nActElecSpd : Inport  Port=2
  s16_uModulDaxQaxVltg : Inport  Port=3
  u16_uSplyVltg : Inport  Port=4
  s16_iActDaxQaxCurr : Inport  Port=5
  enm_stMotoSt : Inport  Port=6
  bol_enPosSCDCalibEnFlg : Inport  Port=7
  u16_phiSensActElecAg : Inport  Port=8
  u8_stMaxFaltLvl : Inport  Port=9
  busOBD_FaltSt : Inport  Port=10
  s16_nFaltRefMechSpd : Inport  Port=11
  s16_trqFaltRefTqLim : Inport  Port=12
  u8_modeMCUOpMode : Inport  Port=13
  u8_tPCBTempSubs : Inport  Port=14
  bol_flgOvrTstCtlUDS2F : Inport  Port=15
  bol_flgPhiSensFaltRawFlg : Inport  Port=16
  u8_FrzFrmSaveFlg : Inport  Port=17
  bol_flgSlepEn : Inport  Port=18
  sss_ASTSlwTaskInHybr : Subsystem  VariantControl=cstHybrCtrlLbl
  sss_ASTSlwTaskInSenl : Subsystem  VariantControl=cstSenlCtrlLbl
  sss_ASTSlwTaskInSens : Subsystem  VariantControl=cstSensCtrlLbl
  busAST_SlwTaskIn : Outport

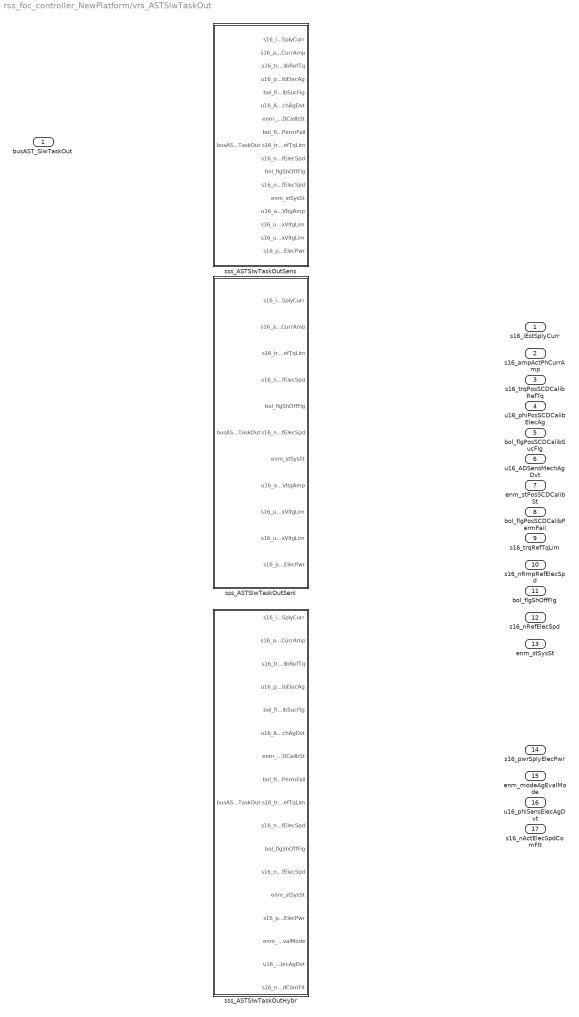
== system rss_foc_controller_NewPlatform/vrs_ASTSlwTaskOut ==
  busAST_SlwTaskOut : Inport
  sss_ASTSlwTaskOutHybr : Subsystem  VariantControl=cstHybrCtrlLbl
  sss_ASTSlwTaskOutSenl : Subsystem  VariantControl=cstSenlCtrlLbl
  sss_ASTSlwTaskOutSens : Subsystem  VariantControl=cstSensCtrlLbl
  s16_iEstSplyCurr : Outport
  s16_ampActPhCurrAmp : Outport  Port=2
  s16_trqPosSCDCalibRefTq : Outport  Port=3
  u16_phiPosSCDCalibElecAg : Outport  Port=4
  bol_flgPosSCDCalibSucFlg : Outport  Port=5
  u16_ADSensMechAgDvt : Outport  Port=6
  enm_stPosSCDCalibSt : Outport  Port=7
  bol_flgPosSCDCalibPermFail : Outport  Port=8
  s16_trqRefTqLim : Outport  Port=9
  s16_nRmpRefElecSpd : Outport  Port=10
  bol_flgShOffFlg : Outport  Port=11
  s16_nRefElecSpd : Outport  Port=12
  enm_stSysSt : Outport  Port=13
  s16_pwrSplyElecPwr : Outport  Port=14
  enm_modeAgEvalMode : Outport  Port=15
  u16_phiSensElecAgDvt : Outport  Port=16
  s16_nActElecSpdComFlt : Outport  Port=17

== system rss_foc_controller_NewPlatform/vrs_DcycGenFstTaskIn ==
  u16_ampDycAmp : Inport
  u16_phiActElecAg : Inport  Port=2
  u16_phiDaxQaxVltgAg : Inport  Port=3
  enm_stMotoSt : Inport  Port=4
  s16_nPredActElecSpd : Inport  Port=5
  bol_enPosSCDCalibEnFlg : Inport  Port=6
  sss_DcycGenFstTaskInSenl : Subsystem  VariantControl=cstSenlCtrlLbl
  sss_DcycGenFstTaskInSens : Subsystem  VariantControl=cstSensCtrlLbl
  busDcycGen_FstTaskIn : Outport  OutDataTypeStr=Bus: BUS_DCYCGEN_FST_TASK_IN

== system rss_foc_controller_NewPlatform/vrs_DcycGenFstTaskOut ==
  busDcycGen_FstTaskOut : Inport
  sss_DcycGenFstTaskOutSenl : Subsystem  VariantControl=cstSenlCtrlLbl
  sss_DcycGenFstTaskOutSens : Subsystem  VariantControl=cstSensCtrlLbl
  u16_dcycPhDyc : Outport  OutDataTypeStr=dt_DutyCycl_u16p15b0
  u16_ampMaxNrmVltgAmp : Outport  Port=2  OutDataTypeStr=dt_DutyCycl_u16p15b0
  u16_phiModulActElecAg : Outport  Port=3  OutDataTypeStr=dt_RadAng_u16r15b0

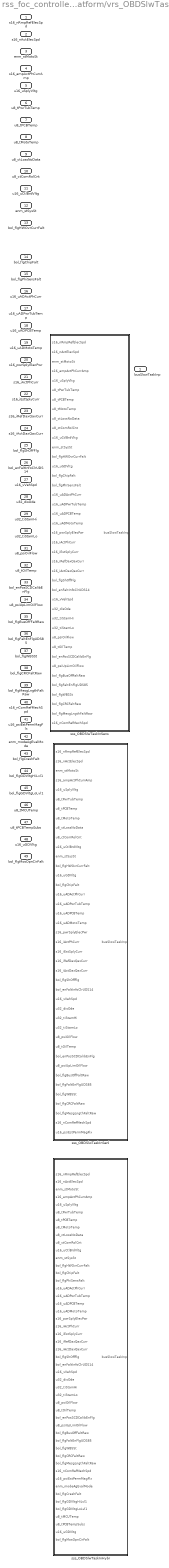
== system rss_foc_controller_NewPlatform/vrs_OBDSlwTaskIn ==
  s16_nRmpRefElecSpd : Inport
  s16_nActElecSpd : Inport  Port=2
  enm_stMotoSt : Inport  Port=3
  s16_ampActPhCurrAmp : Inport  Port=4
  u16_uSplyVltg : Inport  Port=5
  u8_tPwrTubTemp : Inport  Port=6
  u8_tPCBTemp : Inport  Port=7
  u8_tMotoTemp : Inport  Port=8
  u8_ctLossNoData : Inport  Port=9
  u8_ctComRolCnt : Inport  Port=10
  u16_uCtlBrdVltg : Inport  Port=11
  enm_stSysSt : Inport  Port=12
  bol_flgHWOvrCurrFalt : Inport  Port=13
  bol_flgChipFalt : Inport  Port=14
  bol_flgPhiSensFalt : Inport  Port=15
  u16_uADActPhCurr : Inport  Port=16
  u16_uADPwrTubTemp : Inport  Port=17
  u16_uADPCBTemp : Inport  Port=18
  u16_uADMotoTemp : Inport  Port=19
  s16_pwrSplyElecPwr : Inport  Port=20
  s16_iActPhCurr : Inport  Port=21
  s16_iEstSplyCurr : Inport  Port=22
  s16_iRefDaxQaxCurr : Inport  Port=23
  s16_iActDaxQaxCurr : Inport  Port=24
  bol_flgShOffFlg : Inport  Port=25
  bol_enFaltInfoClrUDS14 : Inport  Port=26
  u16_vVehSpd : Inport  Port=27
  u32_disOde : Inport  Port=28
  u32_tiStamHi : Inport  Port=29
  u32_tiStamLo : Inport  Port=30
  u8_psiOilFlow : Inport  Port=31
  u8_tOilTemp : Inport  Port=32
  bol_enPosSCDCalibEnFlg : Inport  Port=33
  u8_psiUpLimOilFlow : Inport  Port=34
  bol_flgBusOffFaltRaw : Inport  Port=35
  bol_flgFaltEnFlgUDS85 : Inport  Port=36
  bol_flgWBSSt : Inport  Port=37
  bol_flgCRCFaltRaw : Inport  Port=38
  bol_flgMesgLngthFaltRaw : Inport  Port=39
  s16_nComRefMechSpd : Inport  Port=40
  u16_psiEstPermMagFlx : Inport  Port=41
  enm_modeAgEvalMode : Inport  Port=42
  bol_flgCrashFalt : Inport  Port=43
  bol_flgGDVltgHiLvl1 : Inport  Port=44
  bol_flgGDVltgLoLvl1 : Inport  Port=45
  u8_tMCUTemp : Inport  Port=46
  u8_tPCBTempSubs : Inport  Port=47
  u16_uGDVltg : Inport  Port=48
  bol_flgMosOpnCirFalt : Inport  Port=49
  sss_OBDSlwTaskInHybr : Subsystem  VariantControl=cstHybrCtrlLbl
  sss_OBDSlwTaskInSenl : Subsystem  VariantControl=cstSenlCtrlLbl
  sss_OBDSlwTaskInSens : Subsystem  VariantControl=cstSensCtrlLbl
  busSlowTaskInp : Outport

== system rss_foc_controller_NewPlatform/vrs_OBDSlwTaskOut ==
  busOBD_SlwTaskOut : Inport
  sss_OBDSlwTaskOutHybr : Subsystem  VariantControl=cstHybrCtrlLbl
  sss_OBDSlwTaskOutSenl : Subsystem  VariantControl=cstSenlCtrlLbl
  sss_OBDSlwTaskOutSens : Subsystem  VariantControl=cstSensCtrlLbl
  busOBD_FaltSt : Outport
  u8_stMaxFaltLvl : Outport  Port=2
  s16_nFaltRefMechSpd : Outport  Port=3
  s16_trqFaltRefTqLim : Outport  Port=4
  bol_flgPhiSensFaltRawFlg : Outport  Port=5

== system rss_foc_controller_NewPlatform/vrs_PhCurrGenSlwTaskIn ==
  s16_nRefElecSpd : Inport
  s16_nActElecSpd : Inport  Port=2
  s16_nRmpRefElecSpd : Inport  Port=3
  s16_trqRefTqLim : Inport  Port=4
  bol_flgShOffFlg : Inport  Port=5
  bol_enPosSCDCalibEnFlg : Inport  Port=6
  s16_trqPosSCDCalibRefTq : Inport  Port=7
  enm_modeAgEvalMode : Inport  Port=8
  s16_phiOpnLpAgClsLpAgDvt : Inport  Port=9
  sss_PhCurrGenSlwTaskInHybr : Subsystem  VariantControl=cstHybrCtrlLbl
  sss_PhCurrGenSlwTaskInSenl : Subsystem  VariantControl=cstSenlCtrlLbl
  sss_PhCurrGenSlwTaskInSens : Subsystem  VariantControl=cstSensCtrlLbl
  busPhCurrGen_SlwTaskIn : Outport

== system rss_foc_controller_NewPlatform/vrs_PhCurrGenSlwTaskOut ==
  busMotoCtl_SlwTaskOut : Inport
  sss_PhCurrGenSlwTaskOutHybr : Subsystem  VariantControl=cstHybrCtrlLbl
  sss_PhCurrGenSlwTaskOutSenl : Subsystem  VariantControl=cstSenlCtrlLbl
  sss_PhCurrGenSlwTaskOutSens : Subsystem  VariantControl=cstSensCtrlLbl
  s16_iRefDaxQaxCurr : Outport
  enm_stMotoSt : Outport  Port=2

== system rss_foc_controller_NewPlatform/vrs_PhVltgGenMedTaskIn ==
  s16_iRefDaxQaxCurr : Inport
  s16_iActPhCurr : Inport  Port=2
  u16_phiSensActElecAg : Inport  Port=3
  u16_uSplyVltg : Inport  Port=4
  enm_stMotoSt : Inport  Port=5
  u16_phiModulActElecAg : Inport  Port=6
  u16_phiPosSCDCalibElecAg : Inport  Port=7  OutDataTypeStr=dt_RadAng_u16r15b0
  u16_dcycPhDyc : Inport  Port=8
  bol_enPosSCDCalibEnFlg : Inport  Port=9
  enm_modeAgEvalMode : Inport  Port=10
  s16_nRmpRefElecSpd : Inport  Port=11
  u8_tPCBTempSubs : Inport  Port=12
  u16_ampMaxNrmVltgAmp : Inport  Port=13
  sss_PhVltgGenMedTaskInHybr : Subsystem  VariantControl=cstHybrCtrlLbl
  sss_PhVltgGenMedTaskInSenl : Subsystem  VariantControl=cstSenlCtrlLbl
  sss_PhVltgGenMedTaskInSens : Subsystem  VariantControl=cstSensCtrlLbl
  busPhVltgGen_MedTaskIn : Outport  OutDataTypeStr=Bus: BUS_PHVLTGGEN_MED_TASK_IN

== system rss_foc_controller_NewPlatform/vrs_PhVltgGenMedTaskOut ==
  busPhVltgGen_MedTaskOut : Inport
  sss_PhVltgGenMedTaskOutHybr : Subsystem  VariantControl=cstHybrCtrlLbl
  sss_PhVltgGenMedTaskOutSenl : Subsystem  VariantControl=cstSenlCtrlLbl
  sss_PhVltgGenMedTaskOutSens : Subsystem  VariantControl=cstSensCtrlLbl
  u16_ampDycAmp : Outport  OutDataTypeStr=dt_DutyCycl_u16p15b0
  u16_phiDaxQaxVltgAg : Outport  Port=2  OutDataTypeStr=dt_RadAng_u16r15b0
  u16_phiActElecAg : Outport  Port=3  OutDataTypeStr=dt_RadAng_u16r15b0
  s16_nActElecSpd : Outport  Port=4  OutDataTypeStr=dt_Standardize_s16p15b0
  s16_iActDaxQaxCurr : Outport  Port=5  OutDataTypeStr=dt_Standardize_s16p15b0
  s16_nPredActElecSpd : Outport  Port=6  OutDataTypeStr=dt_Standardize_s16p15b0
  s16_uModulDaxQaxVltg : Outport  Port=7  OutDataTypeStr=dt_Standardize_s16p15b0
  u16_psiEstPermMagFlx : Outport  Port=8
  s16_phiOpnLpAgClsLpAgDvt : Outport  Port=9

== system rss_foc_controller_NewPlatform/vrs_SigInMedTaskIn ==
  u16_ADSensActMechAg : Inport
  u16_uADActPhCurr : Inport  Port=2
  u16_uADActPhCurrOfs : Inport  Port=3
  u8_numSectNum : Inport  Port=4
  u16_uADSplyVltg : Inport  Port=5
  u16_phiDvtSensElecAg : Inport  Port=6
  bol_enPosSCDCalibEnFlg : Inport  Port=7
  sss_SigInMedTaskInSenl : Subsystem  VariantControl=cstSenlCtrlLbl
  sss_SigInMedTaskInSens : Subsystem  VariantControl=cstSensCtrlLbl
  busSigIn_MedTaskIn : Outport

== system rss_foc_controller_NewPlatform/vrs_SigInMedTaskOut ==
  busSigIn_MedTaskOut : Inport
  sss_SigInMedTaskOutHybr : Subsystem  VariantControl=cstHybrCtrlLbl
  sss_SigInMedTaskOutSenl : Subsystem  VariantControl=cstSenlCtrlLbl
  sss_SigInMedTaskOutSens : Subsystem  VariantControl=cstSensCtrlLbl
  u16_phiSensActElecAg : Outport
  s16_iActPhCurr : Outport  Port=2
  u16_uSplyVltg : Outport  Port=3

== system rss_foc_controller_NewPlatform/vrs_SigInSlwTaskOut ==
  busSigIn_SlwTaskOut : Inport
  sss_SigInSlwTaskOutHybr : Subsystem  VariantControl=cstHybrCtrlLbl
  sss_SigInSlwTaskOutSenl : Subsystem  VariantControl=cstSenlCtrlLbl
  sss_SigInSlwTaskOutSens : Subsystem  VariantControl=cstSensCtrlLbl
  u16_uCtlBrdVltg : Outport
  u16_uGDVltg : Outport  Port=2
  u8_tPwrTubTemp : Outport  Port=3
  u8_tPCBTemp : Outport  Port=4
  u8_tMotoTemp : Outport  Port=5
  u8_tPCBTempSubs : Outport  Port=6

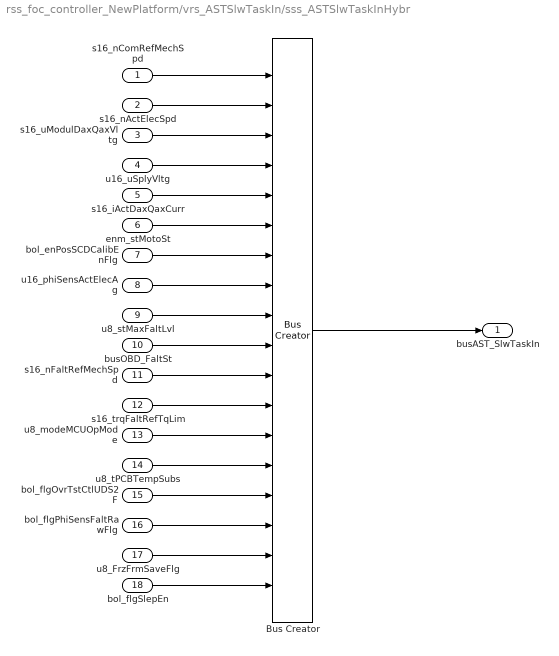
== system rss_foc_controller_NewPlatform/vrs_ASTSlwTaskIn/sss_ASTSlwTaskInHybr ==
  s16_nComRefMechSpd : Inport
  s16_nActElecSpd : Inport  Port=2
  s16_uModulDaxQaxVltg : Inport  Port=3
  u16_uSplyVltg : Inport  Port=4
  s16_iActDaxQaxCurr : Inport  Port=5
  enm_stMotoSt : Inport  Port=6
  bol_enPosSCDCalibEnFlg : Inport  Port=7
  u16_phiSensActElecAg : Inport  Port=8
  u8_stMaxFaltLvl : Inport  Port=9
  busOBD_FaltSt : Inport  Port=10
  s16_nFaltRefMechSpd : Inport  Port=11
  s16_trqFaltRefTqLim : Inport  Port=12
  u8_modeMCUOpMode : Inport  Port=13
  u8_tPCBTempSubs : Inport  Port=14
  bol_flgOvrTstCtlUDS2F : Inport  Port=15
  bol_flgPhiSensFaltRawFlg : Inport  Port=16
  u8_FrzFrmSaveFlg : Inport  Port=17
  bol_flgSlepEn : Inport  Port=18
  Bus Creator : BusCreator  Inputs=18  OutDataTypeStr=Bus: BUS_AST_SLW_TASK_IN
      settings: InheritFromInputs=off
  busAST_SlwTaskIn : Outport  OutDataTypeStr=Bus: BUS_AST_SLW_TASK_IN
  wires:
  bol_flgPhiSensFaltRawFlg/1 -> Bus Creator/16
  bol_flgOvrTstCtlUDS2F/1 -> Bus Creator/15
  bol_flgSlepEn/1 -> Bus Creator/18
  u8_FrzFrmSaveFlg/1 -> Bus Creator/17
  u8_tPCBTempSubs/1 -> Bus Creator/14
  u8_modeMCUOpMode/1 -> Bus Creator/13
  bol_enPosSCDCalibEnFlg/1 -> Bus Creator/7
  s16_trqFaltRefTqLim/1 -> Bus Creator/12
  s16_nFaltRefMechSpd/1 -> Bus Creator/11
  busOBD_FaltSt/1 -> Bus Creator/10
  u8_stMaxFaltLvl/1 -> Bus Creator/9
  u16_phiSensActElecAg/1 -> Bus Creator/8
  s16_nComRefMechSpd/1 -> Bus Creator/1
  s16_nActElecSpd/1 -> Bus Creator/2
  s16_uModulDaxQaxVltg/1 -> Bus Creator/3
  u16_uSplyVltg/1 -> Bus Creator/4
  s16_iActDaxQaxCurr/1 -> Bus Creator/5
  enm_stMotoSt/1 -> Bus Creator/6
  Bus Creator/1 -> busAST_SlwTaskIn/1

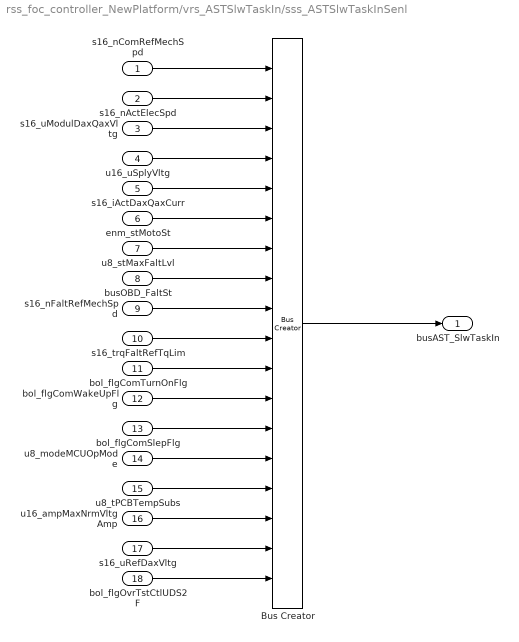
== system rss_foc_controller_NewPlatform/vrs_ASTSlwTaskIn/sss_ASTSlwTaskInSenl ==
  s16_nComRefMechSpd : Inport
  s16_nActElecSpd : Inport  Port=2
  s16_uModulDaxQaxVltg : Inport  Port=3
  u16_uSplyVltg : Inport  Port=4
  s16_iActDaxQaxCurr : Inport  Port=5
  enm_stMotoSt : Inport  Port=6
  u8_stMaxFaltLvl : Inport  Port=7
  busOBD_FaltSt : Inport  Port=8
  s16_nFaltRefMechSpd : Inport  Port=9
  s16_trqFaltRefTqLim : Inport  Port=10
  bol_flgComTurnOnFlg : Inport  Port=11
  bol_flgComWakeUpFlg : Inport  Port=12
  bol_flgComSlepFlg : Inport  Port=13
  u8_modeMCUOpMode : Inport  Port=14
  u8_tPCBTempSubs : Inport  Port=15
  u16_ampMaxNrmVltgAmp : Inport  Port=16
  s16_uRefDaxVltg : Inport  Port=17
  bol_flgOvrTstCtlUDS2F : Inport  Port=18
  Bus Creator : BusCreator  Inputs=18  OutDataTypeStr=Bus: BUS_AST_SLW_TASK_IN
      settings: InheritFromInputs=off
  busAST_SlwTaskIn : Outport  OutDataTypeStr=Bus: BUS_AST_SLW_TASK_IN
  wires:
  bol_flgOvrTstCtlUDS2F/1 -> Bus Creator/18
  s16_uRefDaxVltg/1 -> Bus Creator/17
  u16_ampMaxNrmVltgAmp/1 -> Bus Creator/16
  u8_tPCBTempSubs/1 -> Bus Creator/15
  u8_modeMCUOpMode/1 -> Bus Creator/14
  bol_flgComSlepFlg/1 -> Bus Creator/13
  bol_flgComWakeUpFlg/1 -> Bus Creator/12
  bol_flgComTurnOnFlg/1 -> Bus Creator/11
  s16_trqFaltRefTqLim/1 -> Bus Creator/10
  s16_nFaltRefMechSpd/1 -> Bus Creator/9
  busOBD_FaltSt/1 -> Bus Creator/8
  u8_stMaxFaltLvl/1 -> Bus Creator/7
  Bus Creator/1 -> busAST_SlwTaskIn/1
  enm_stMotoSt/1 -> Bus Creator/6
  s16_iActDaxQaxCurr/1 -> Bus Creator/5
  u16_uSplyVltg/1 -> Bus Creator/4
  s16_uModulDaxQaxVltg/1 -> Bus Creator/3
  s16_nActElecSpd/1 -> Bus Creator/2
  s16_nComRefMechSpd/1 -> Bus Creator/1

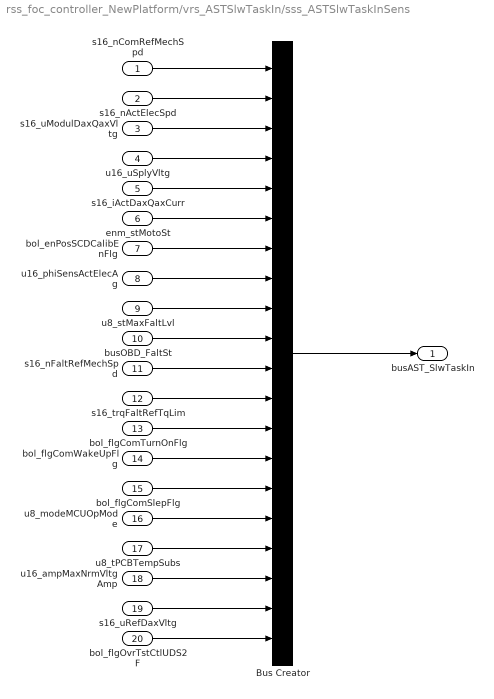
== system rss_foc_controller_NewPlatform/vrs_ASTSlwTaskIn/sss_ASTSlwTaskInSens ==
  s16_nComRefMechSpd : Inport
  s16_nActElecSpd : Inport  Port=2
  s16_uModulDaxQaxVltg : Inport  Port=3
  u16_uSplyVltg : Inport  Port=4
  s16_iActDaxQaxCurr : Inport  Port=5
  enm_stMotoSt : Inport  Port=6
  bol_enPosSCDCalibEnFlg : Inport  Port=7
  u16_phiSensActElecAg : Inport  Port=8
  u8_stMaxFaltLvl : Inport  Port=9
  busOBD_FaltSt : Inport  Port=10
  s16_nFaltRefMechSpd : Inport  Port=11
  s16_trqFaltRefTqLim : Inport  Port=12
  bol_flgComTurnOnFlg : Inport  Port=13
  bol_flgComWakeUpFlg : Inport  Port=14
  bol_flgComSlepFlg : Inport  Port=15
  u8_modeMCUOpMode : Inport  Port=16
  u8_tPCBTempSubs : Inport  Port=17
  u16_ampMaxNrmVltgAmp : Inport  Port=18
  s16_uRefDaxVltg : Inport  Port=19
  bol_flgOvrTstCtlUDS2F : Inport  Port=20
  Bus Creator : BusCreator  Inputs=20  OutDataTypeStr=Bus: BUS_AST_SLW_TASK_IN
      settings: InheritFromInputs=off
  busAST_SlwTaskIn : Outport  OutDataTypeStr=Bus: BUS_AST_SLW_TASK_IN
  wires:
  bol_flgOvrTstCtlUDS2F/1 -> Bus Creator/20
  Bus Creator/1 -> busAST_SlwTaskIn/1
  s16_uRefDaxVltg/1 -> Bus Creator/19
  u16_ampMaxNrmVltgAmp/1 -> Bus Creator/18
  u8_tPCBTempSubs/1 -> Bus Creator/17
  u8_modeMCUOpMode/1 -> Bus Creator/16
  bol_flgComSlepFlg/1 -> Bus Creator/15
  bol_flgComWakeUpFlg/1 -> Bus Creator/14
  bol_flgComTurnOnFlg/1 -> Bus Creator/13
  s16_trqFaltRefTqLim/1 -> Bus Creator/12
  s16_nFaltRefMechSpd/1 -> Bus Creator/11
  busOBD_FaltSt/1 -> Bus Creator/10
  u8_stMaxFaltLvl/1 -> Bus Creator/9
  u16_phiSensActElecAg/1 -> Bus Creator/8
  bol_enPosSCDCalibEnFlg/1 -> Bus Creator/7
  enm_stMotoSt/1 -> Bus Creator/6
  s16_iActDaxQaxCurr/1 -> Bus Creator/5
  u16_uSplyVltg/1 -> Bus Creator/4
  s16_uModulDaxQaxVltg/1 -> Bus Creator/3
  s16_nActElecSpd/1 -> Bus Creator/2
  s16_nComRefMechSpd/1 -> Bus Creator/1

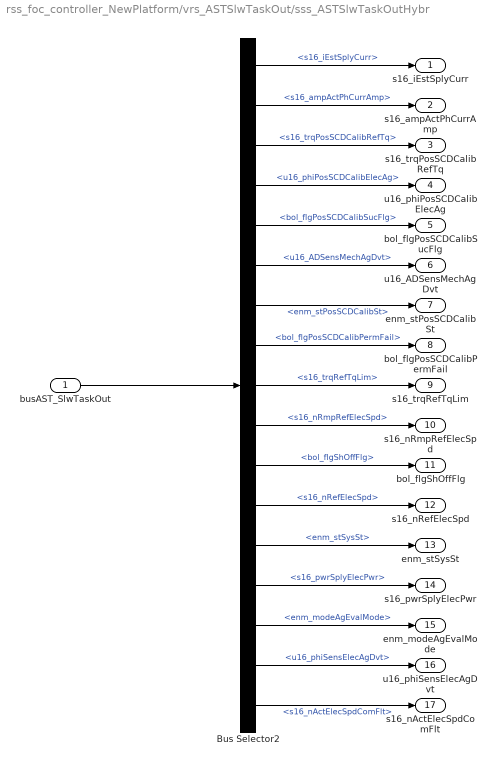
== system rss_foc_controller_NewPlatform/vrs_ASTSlwTaskOut/sss_ASTSlwTaskOutHybr ==
  busAST_SlwTaskOut : Inport
  Bus Selector2 : BusSelector  OutputSignals=s16_iEstSplyCurr,s16_ampActPhCurrAmp,s16_trqPosSCDCalibRefTq,u16_phiPosSCDCalibElecAg,bol_flgPosSCDCalibSucFlg,u16_ADSensMechAgDvt,enm_stPosSCDCalibSt,bol_flgPosSCDCalibPermFail,s16_trqRefTqLim,s16_nRmpRefElecSpd,bol_flgShOffFlg,s16_nRefElecSpd,enm_stSysSt,s16_pwrSplyElecPwr,enm_modeAgEvalMode,u16_phiSensElecAgDvt,s16_nActElecSpdComFlt
  s16_iEstSplyCurr : Outport
  s16_ampActPhCurrAmp : Outport  Port=2
  s16_trqPosSCDCalibRefTq : Outport  Port=3
  u16_phiPosSCDCalibElecAg : Outport  Port=4
  bol_flgPosSCDCalibSucFlg : Outport  Port=5
  u16_ADSensMechAgDvt : Outport  Port=6
  enm_stPosSCDCalibSt : Outport  Port=7
  bol_flgPosSCDCalibPermFail : Outport  Port=8
  s16_trqRefTqLim : Outport  Port=9
  s16_nRmpRefElecSpd : Outport  Port=10
  bol_flgShOffFlg : Outport  Port=11
  s16_nRefElecSpd : Outport  Port=12
  enm_stSysSt : Outport  Port=13
  s16_pwrSplyElecPwr : Outport  Port=14
  enm_modeAgEvalMode : Outport  Port=15
  u16_phiSensElecAgDvt : Outport  Port=16
  s16_nActElecSpdComFlt : Outport  Port=17
  wires:
  Bus Selector2/17 -> s16_nActElecSpdComFlt/1  "<s16_nActElecSpdComFlt>"
  Bus Selector2/16 -> u16_phiSensElecAgDvt/1  "<u16_phiSensElecAgDvt>"
  Bus Selector2/8 -> bol_flgPosSCDCalibPermFail/1  "<bol_flgPosSCDCalibPermFail>"
  Bus Selector2/7 -> enm_stPosSCDCalibSt/1  "<enm_stPosSCDCalibSt>"
  Bus Selector2/6 -> u16_ADSensMechAgDvt/1  "<u16_ADSensMechAgDvt>"
  Bus Selector2/5 -> bol_flgPosSCDCalibSucFlg/1  "<bol_flgPosSCDCalibSucFlg>"
  Bus Selector2/4 -> u16_phiPosSCDCalibElecAg/1  "<u16_phiPosSCDCalibElecAg>"
  Bus Selector2/3 -> s16_trqPosSCDCalibRefTq/1  "<s16_trqPosSCDCalibRefTq>"
  Bus Selector2/15 -> enm_modeAgEvalMode/1  "<enm_modeAgEvalMode>"
  Bus Selector2/13 -> enm_stSysSt/1  "<enm_stSysSt>"
  Bus Selector2/14 -> s16_pwrSplyElecPwr/1  "<s16_pwrSplyElecPwr>"
  Bus Selector2/11 -> bol_flgShOffFlg/1  "<bol_flgShOffFlg>"
  Bus Selector2/12 -> s16_nRefElecSpd/1  "<s16_nRefElecSpd>"
  Bus Selector2/2 -> s16_ampActPhCurrAmp/1  "<s16_ampActPhCurrAmp>"
  Bus Selector2/1 -> s16_iEstSplyCurr/1  "<s16_iEstSplyCurr>"
  Bus Selector2/10 -> s16_nRmpRefElecSpd/1  "<s16_nRmpRefElecSpd>"
  Bus Selector2/9 -> s16_trqRefTqLim/1  "<s16_trqRefTqLim>"
  busAST_SlwTaskOut/1 -> Bus Selector2/1

== system rss_foc_controller_NewPlatform/vrs_ASTSlwTaskOut/sss_ASTSlwTaskOutSenl ==
  busAST_SlwTaskOut : Inport
  Bus Selector2 : BusSelector  OutputSignals=s16_iEstSplyCurr,s16_ampActPhCurrAmp,s16_trqRefTqLim,s16_nRmpRefElecSpd,bol_flgShOffFlg,s16_nRefElecSpd,enm_stSysSt,u16_ampMaxVltgAmp,s16_uRefDaxVltgLim,s16_uRefQaxVltgLim,s16_pwrSplyElecPwr
  s16_iEstSplyCurr : Outport
  s16_ampActPhCurrAmp : Outport  Port=2
  s16_trqRefTqLim : Outport  Port=3
  s16_nRmpRefElecSpd : Outport  Port=4
  bol_flgShOffFlg : Outport  Port=5
  s16_nRefElecSpd : Outport  Port=6
  enm_stSysSt : Outport  Port=7
  u16_ampMaxVltgAmp : Outport  Port=8
  s16_uRefDaxVltgLim : Outport  Port=9
  s16_uRefQaxVltgLim : Outport  Port=10
  s16_pwrSplyElecPwr : Outport  Port=11
  wires:
  Bus Selector2/11 -> s16_pwrSplyElecPwr/1  "<s16_pwrSplyElecPwr>"
  busAST_SlwTaskOut/1 -> Bus Selector2/1
  Bus Selector2/1 -> s16_iEstSplyCurr/1  "<s16_iEstSplyCurr>"
  Bus Selector2/8 -> u16_ampMaxVltgAmp/1  "<u16_ampMaxVltgAmp>"
  Bus Selector2/4 -> s16_nRmpRefElecSpd/1  "<s16_nRmpRefElecSpd>"
  Bus Selector2/3 -> s16_trqRefTqLim/1  "<s16_trqRefTqLim>"
  Bus Selector2/7 -> enm_stSysSt/1  "<enm_stSysSt>"
  Bus Selector2/2 -> s16_ampActPhCurrAmp/1  "<s16_ampActPhCurrAmp>"
  Bus Selector2/5 -> bol_flgShOffFlg/1  "<bol_flgShOffFlg>"
  Bus Selector2/10 -> s16_uRefQaxVltgLim/1  "<s16_uRefQaxVltgLim>"
  Bus Selector2/6 -> s16_nRefElecSpd/1  "<s16_nRefElecSpd>"
  Bus Selector2/9 -> s16_uRefDaxVltgLim/1  "<s16_uRefDaxVltgLim>"

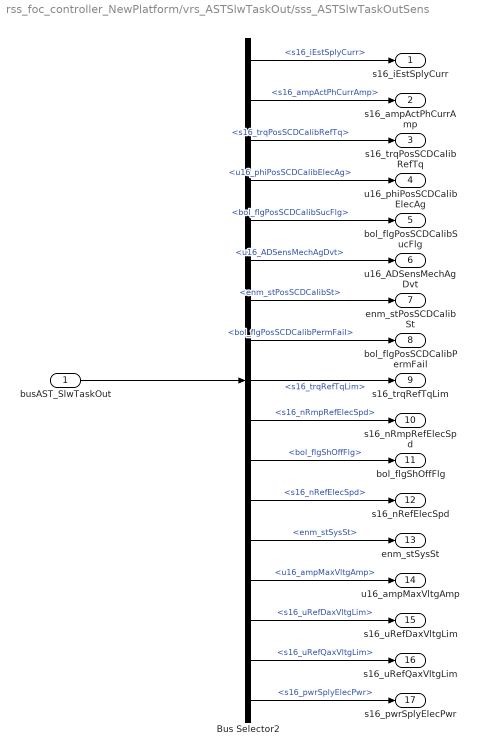
== system rss_foc_controller_NewPlatform/vrs_ASTSlwTaskOut/sss_ASTSlwTaskOutSens ==
  busAST_SlwTaskOut : Inport
  Bus Selector2 : BusSelector  OutputSignals=s16_iEstSplyCurr,s16_ampActPhCurrAmp,s16_trqPosSCDCalibRefTq,u16_phiPosSCDCalibElecAg,bol_flgPosSCDCalibSucFlg,u16_ADSensMechAgDvt,enm_stPosSCDCalibSt,bol_flgPosSCDCalibPermFail,s16_trqRefTqLim,s16_nRmpRefElecSpd,bol_flgShOffFlg,s16_nRefElecSpd,enm_stSysSt,u16_ampMaxVltgAmp,s16_uRefDaxVltgLim,s16_uRefQaxVltgLim,s16_pwrSplyElecPwr
  s16_iEstSplyCurr : Outport
  s16_ampActPhCurrAmp : Outport  Port=2
  s16_trqPosSCDCalibRefTq : Outport  Port=3
  u16_phiPosSCDCalibElecAg : Outport  Port=4
  bol_flgPosSCDCalibSucFlg : Outport  Port=5
  u16_ADSensMechAgDvt : Outport  Port=6
  enm_stPosSCDCalibSt : Outport  Port=7
  bol_flgPosSCDCalibPermFail : Outport  Port=8
  s16_trqRefTqLim : Outport  Port=9
  s16_nRmpRefElecSpd : Outport  Port=10
  bol_flgShOffFlg : Outport  Port=11
  s16_nRefElecSpd : Outport  Port=12
  enm_stSysSt : Outport  Port=13
  u16_ampMaxVltgAmp : Outport  Port=14
  s16_uRefDaxVltgLim : Outport  Port=15
  s16_uRefQaxVltgLim : Outport  Port=16
  s16_pwrSplyElecPwr : Outport  Port=17
  wires:
  Bus Selector2/17 -> s16_pwrSplyElecPwr/1  "<s16_pwrSplyElecPwr>"
  Bus Selector2/16 -> s16_uRefQaxVltgLim/1  "<s16_uRefQaxVltgLim>"
  Bus Selector2/15 -> s16_uRefDaxVltgLim/1  "<s16_uRefDaxVltgLim>"
  Bus Selector2/14 -> u16_ampMaxVltgAmp/1  "<u16_ampMaxVltgAmp>"
  Bus Selector2/13 -> enm_stSysSt/1  "<enm_stSysSt>"
  Bus Selector2/12 -> s16_nRefElecSpd/1  "<s16_nRefElecSpd>"
  Bus Selector2/11 -> bol_flgShOffFlg/1  "<bol_flgShOffFlg>"
  Bus Selector2/10 -> s16_nRmpRefElecSpd/1  "<s16_nRmpRefElecSpd>"
  Bus Selector2/9 -> s16_trqRefTqLim/1  "<s16_trqRefTqLim>"
  Bus Selector2/8 -> bol_flgPosSCDCalibPermFail/1  "<bol_flgPosSCDCalibPermFail>"
  Bus Selector2/7 -> enm_stPosSCDCalibSt/1  "<enm_stPosSCDCalibSt>"
  Bus Selector2/6 -> u16_ADSensMechAgDvt/1  "<u16_ADSensMechAgDvt>"
  Bus Selector2/5 -> bol_flgPosSCDCalibSucFlg/1  "<bol_flgPosSCDCalibSucFlg>"
  Bus Selector2/4 -> u16_phiPosSCDCalibElecAg/1  "<u16_phiPosSCDCalibElecAg>"
  Bus Selector2/3 -> s16_trqPosSCDCalibRefTq/1  "<s16_trqPosSCDCalibRefTq>"
  Bus Selector2/2 -> s16_ampActPhCurrAmp/1  "<s16_ampActPhCurrAmp>"
  Bus Selector2/1 -> s16_iEstSplyCurr/1  "<s16_iEstSplyCurr>"
  busAST_SlwTaskOut/1 -> Bus Selector2/1
